simulink model "Model"  (R2024b)
settings: Solver=VariableStepAuto  StartTime=0.0  StopTime=10.0  RelTol=1e-3
undefined symbols (not defined in the file): b, J, K, L, R
libraries: slpidlib x1
settings Model: Creator=Eng.Ahmed  LastModifiedBy=Eng.Ahmed

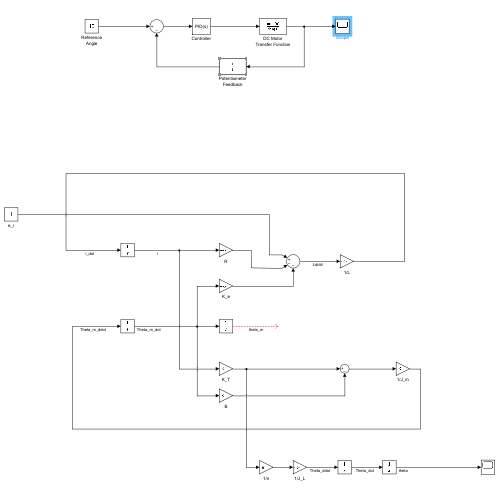
[thumbnail: Simulink's stored preview of the top-level diagram]
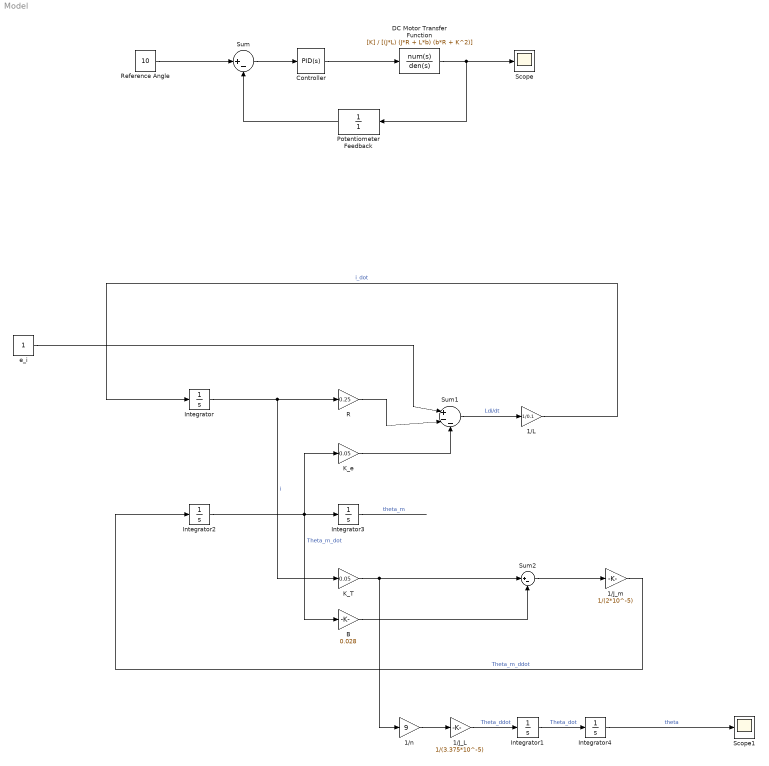
== system Model ==
  1/J_L : Gain  Gain=1/(3.375*10^-5)
  1/J_m : Gain  Gain=1/(2*10^-5)
  1/L : Gain  Gain=1/0.1
  1/n : Gain  Gain=9
  B : Gain  Gain=0.028
  Controller : slpidlib/PID Controller  Controller=PID  Form=Parallel  TimeDomain=Continuous-time  UseExternalTs=off  SampleTime=-1  IntegratorMethod=Forward Euler  FilterMethod=Forward Euler  ControllerParametersSource=internal  P=1.835  I=0.5  UseKiTs=off  D=0.8835  UseExternalDerivativeSource=off  N=100  UseFilter=on  TunerSelectOption=Transfer Function Based (PID Tuner App)  InitialConditionSource=internal  InitialConditionForIntegrator=0  InitialConditionForFilter=0  DifferentiatorICPrevScaledInput=0  ExternalReset=none  TrackingMode=off  Kt=1  LimitOutput=off  SatLimitsSource=internal  UpperSaturationLimit=inf  LowerSaturationLimit=-inf  LinearizeAsGain=on  AntiWindupMode=none  Kb=1  LimitIntegrator=off  UpperIntegratorSaturationLimit=inf  LowerIntegratorSaturationLimit=-inf  POutMin=[]  POutMax=[]  IOutMin=[]  IOutMax=[]  DOutMin=[]  DOutMax=[]  NOutMin=[]  NOutMax=[]  SumOutMin=[]  SumOutMax=[]  SaturationOutMin=[]  SaturationOutMax=[]  PParamMin=[]  PParamMax=[]  IParamMin=[]  IParamMax=[]  DParamMin=[]  DParamMax=[]  NParamMin=[]  NParamMax=[]  KbParamMin=[]  KbParamMax=[]  KtParamMin=[]  KtParamMax=[]  KbOutMin=[]  KbOutMax=[]  KtOutMin=[]  KtOutMax=[]  IntegratorOutMin=[]  IntegratorOutMax=[]  FilterOutMin=[]  FilterOutMax=[]  SumI1OutMin=[]  SumI1OutMax=[]  SumI2OutMin=[]  SumI2OutMax=[]  SumI3OutMin=[]  SumI3OutMax=[]  SumI4OutMin=[]  SumI4OutMax=[]  SumDOutMin=[]  SumDOutMax=[]  DifferentiatorOutMin=[]  DifferentiatorOutMax=[]  FilterDiffOutCoefMin=[]  FilterDiffOutCoefMax=[]  ReciprocalOutMin=[]  ReciprocalOutMax=[]  SumDenOutMin=[]  SumDenOutMax=[]  SumNumOutMin=[]  SumNumOutMax=[]  DivideOutMin=[]  DivideOutMax=[]  UdiffTsProdOutMin=[]  UdiffTsProdOutMax=[]  NTsProdOutMin=[]  NTsProdOutMax=[]  UintegralTsProdOutMin=[]  UintegralTsProdOutMax=[]  UngainTsProdOutMin=[]  UngainTsProdOutMax=[]  ClampingZeroOutDataTypeStr=Inherit: Inherit via back propagation  ClampingZeroOutMin=[]  ClampingZeroOutMax=[]  FilterDenConstantOutDataTypeStr=Inherit: Inherit via back propagation  FilterDenConstantOutMin=[]  FilterDenConstantOutMax=[]  PCopyOutDataTypeStr=Inherit: Inherit via back propagation  PCopyOutMin=[]  PCopyOutMax=[]  NCopyOutDataTypeStr=Inherit: Inherit via back propagation  NCopyOutMin=[]  NCopyOutMax=[]  IntegratorContinuousStateAttributes=''  IntegratorStateMustResolveToSignalObject=off  IntegratorRTWStateStorageClass=Auto  FilterContinuousStateAttributes=''  FilterStateMustResolveToSignalObject=off  FilterRTWStateStorageClass=Auto  ParallelPVariant=InternalParameters  IdealPVariant=Disabled  IVariant=InternalParameters  DVariant=InternalParameters  IntegratorVariant=Continuous  SatVariant=Disabled  AWVariant=Passthrough  PCopyVariant=Disabled  TRVariant=Disabled  FdbkBlocksVariant=Forward  IdealPFdbkVariant=Disabled  SatFdbkVariant=Disabled  DerivativeFilterVariant=ContFilter  NVariant=InternalParameters  NCopyVariant=Disabled  FilterICVariant=InternalICsFilter  IntegratorICVariant=InternalICs  ExternalResetVariant=Disabled  TRSumVariant=Passthrough  SumFdbkVariant=Disabled  SumVariant=Sum_PID  TsampFilterVariant=InternalTs  TsampNgainVariant=Passthrough  TsampIntegralVariant=Disabled_SignalSpec  ExternalSaturationOutDataTypeStr=Inherit: Same as second input  DerivativeSourceVariant=ErrorSignal  PreIntVariant=InternalPreInt
  DC Motor Transfer Function : TransferFcn  Numerator=[K]  Denominator=[(J*L) (J*R + L*b) (b*R + K^2)]
  Integrator{,1..4} (5 alike) : Integrator
  K_T : Gain  Gain=0.05
  K_e : Gain  Gain=0.05
  Potentiometer Feedback : TransferFcn  Denominator=[1]
  R : Gain  Gain=0.25
  Reference Angle : Constant  Value=10
  Scope : Scope
  Scope1 : Scope
  Sum : Sum  Inputs=|+-
  Sum1 : Sum  Inputs=|+--
  Sum2 : Sum  Inputs=|+-
  e_i : Constant
  wires:
  Reference Angle/1 -> Sum/1
  Sum/1 -> Controller/1
  DC Motor Transfer Function/1 -> Potentiometer Feedback/1, Scope/1
  Potentiometer Feedback/1 -> Sum/2
  Integrator3/1 -> ?  "theta_m"
  1/n/1 -> 1/J_L/1
  e_i/1 -> Sum1/1
  1/J_L/1 -> Integrator1/1  "Theta_ddot"
  1/J_m/1 -> Integrator2/1  "Theta_m_ddot"
  Integrator/1 -> R/1, K_T/1  "i"
  B/1 -> Sum2/2
  Integrator2/1 -> B/1, K_e/1, Integrator3/1  "Theta_m_dot"
  Integrator1/1 -> Integrator4/1  "Theta_dot"
  K_e/1 -> Sum1/3
  Sum2/1 -> 1/J_m/1
  1/L/1 -> Integrator/1  "i_dot"
  Integrator4/1 -> Scope1/1  "theta"
  Sum1/1 -> 1/L/1  "Ldi/dt"
  K_T/1 -> 1/n/1, Sum2/1
  R/1 -> Sum1/2
  Controller/1 -> DC Motor Transfer Function/1
